simulink model "Problem_No2"  (R2020a)
settings: Solver=VariableStepAuto  StartTime=0.0  StopTime=10.0  MaxStep=1  RelTol=1e-3
model workspace (MAT data in the model file):
  b = 1000
  k1 = 36000
  k2 = 204034.4
  m1 = 600
  m2 = 90
settings Model: Creator='Z'ome  LastModifiedBy='Z'ome

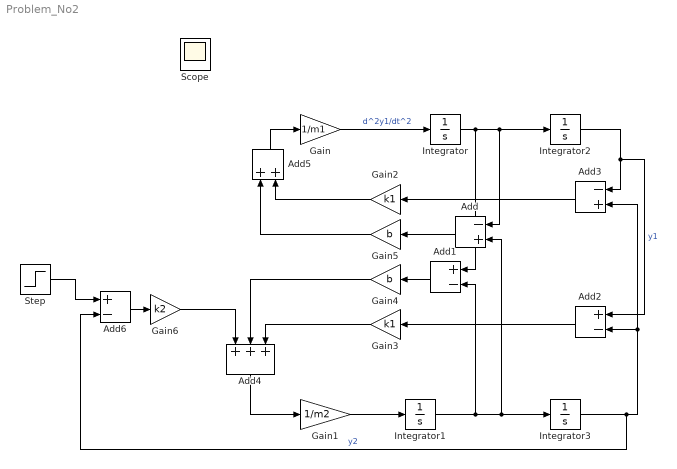
== system Problem_No2 ==
  Add : Sum  Inputs=-+
  Add1 : Sum  Inputs=+-
  Add2 : Sum  Inputs=+-
  Add3 : Sum  Inputs=-+
  Add4 : Sum  Inputs=+++
  Add5 : Sum
  Add6 : Sum  Inputs=+-
  Gain : Gain  Gain=1/m1
  Gain1 : Gain  Gain=1/m2
  Gain2 : Gain  Gain=k1
  Gain3 : Gain  Gain=k1
  Gain4 : Gain  Gain=b
  Gain5 : Gain  Gain=b
  Gain6 : Gain  Gain=k2
  Integrator{,1..3} (4 alike) : Integrator
  Step : Step  SampleTime=0
  Scope : Scope
  wires:
  Gain/1 -> Integrator/1  "d^2y1/dt^2"
  Integrator1/1 -> Add1/2, Add/2, Integrator3/1
  Gain1/1 -> Integrator1/1
  Integrator/1 -> Add1/1, Add/1, Integrator2/1
  Add/1 -> Gain5/1
  Add1/1 -> Gain4/1
  Add2/1 -> Gain3/1
  Add3/1 -> Gain2/1
  Integrator2/1 -> Add2/1, Add3/1  "y1"
  Integrator3/1 -> Add6/2, Add2/2, Add3/2  "y2"
  Add5/1 -> Gain/1
  Gain2/1 -> Add5/2
  Gain5/1 -> Add5/1
  Gain3/1 -> Add4/3
  Gain4/1 -> Add4/2
  Add4/1 -> Gain1/1
  Gain6/1 -> Add4/1
  Add6/1 -> Gain6/1
  Step/1 -> Add6/1
